simulink subsystem "tractionControl"  (R2022b)
settings: Solver=VariableStepAuto  StartTime=0.0  StopTime=10.0  RelTol=1e-3
libraries: Raptor_lib x1, tractionControl_lib x1
settings Model: Creator=serga  LastModifiedBy=serga

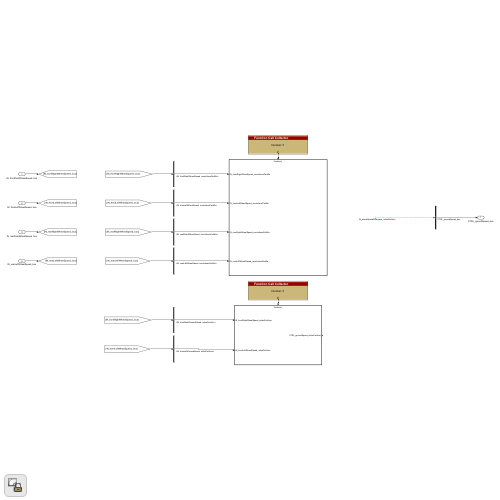
[thumbnail: Simulink's stored preview of the top-level diagram]
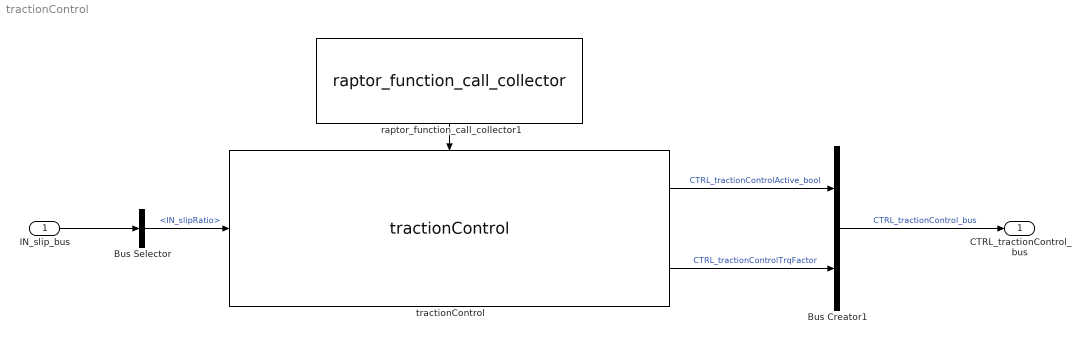
== system tractionControl ==
  IN_slip_bus : Inport
  Bus Creator1 : BusCreator  Inputs=2
  Bus Selector : BusSelector  OutputSignals=IN_slipRatio
  raptor_function_call_collector1 : Raptor_lib/Triggers/raptor_function_call_collector  count=5
      settings: SourceProductName=Raptor
  tractionControl : tractionControl_lib/tractionControl  SystemSampleTime=-1  VariantActivationTime=update diagram  Latency=0  AutoFrameSizeCalculation=off
  CTRL_tractionControl_bus : Outport
  wires:
  raptor_function_call_collector1/1 -> tractionControl/Trigger
  IN_slip_bus/1 -> Bus Selector/1
  Bus Selector/1 -> tractionControl/1  "<IN_slipRatio>"
  tractionControl/2 -> Bus Creator1/2  "CTRL_tractionControlTrqFactor"
  tractionControl/1 -> Bus Creator1/1  "CTRL_tractionControlActive_bool"
  Bus Creator1/1 -> CTRL_tractionControl_bus/1  "CTRL_tractionControl_bus"
